simulink model "Levitatore_dee_mdl"  (Simulink 7.5)
settings: Solver=ode45  StartTime=0.0  StopTime=10.0  MaxStep=1e-2  RelTol=1e-3
values from neighbouring files (symbols this model uses):
  g = 9.81    [TSC160127ProvaMatlab.m]
  k0 = 4    [TSC160127ProvaMatlab.m]
  km = 5    [TSC160127ProvaMatlab.m]
  kv = 1    [TSC160127ProvaMatlab.m]
  m = 5    [TSC160127ProvaMatlab.m]
  v0 = 2    [TSC160127ProvaMatlab.m]
settings Model: Creator=lbiagiotti  LastModifiedBy=Biagio
settings DebuggingCC: StrictBusMsg=Warning

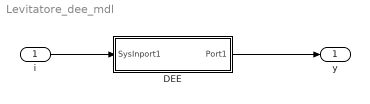
== system Levitatore_dee_mdl ==
  i : Inport  OutDataType=sfix(16)  OutScaling=2^0
  DEE : Subsystem
      settings: OpenFcn=diffeqed
      mask Type: Differential Equation Editor (DEE)
      mask Display: disp('Levitatore')
  y : Outport  OutDataType=sfix(16)  OutScaling=2^0
  wires:
  i/1 -> DEE/1(SysInport1)
  DEE/1(Port1) -> y/1

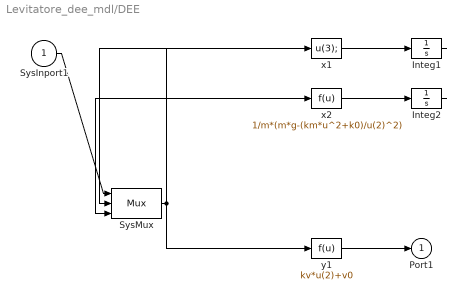
== system Levitatore_dee_mdl/DEE ==
  SysInport1 : Inport
  Integ1 : Integrator  InitialCondition=1
  Integ2 : Integrator
  SysMux : Mux  Inputs=3
  x1 : Fcn  Expr=u(3);
  x2 : Fcn  Expr=1/m*(m*g-(km*u^2+k0)/u(2)^2)
  y1 : Fcn  Expr=kv*u(2)+v0
  Port1 : Outport
  wires:
  SysInport1/1 -> SysMux/1
  SysMux/1 -> x1/1, x2/1, y1/1
  x1/1 -> Integ1/1
  Integ1/1 -> SysMux/2
  x2/1 -> Integ2/1
  Integ2/1 -> SysMux/3
  y1/1 -> Port1/1
